simulink library "F3M_aqueousLib"  (R2023b)
settings: Solver=VariableStepAuto  StartTime=0.0  StopTime=10.0  RelTol=1e-3
undefined symbols (not defined in the file): entity, F3_getArrayPos, F3_ptableToFlow, F3_ptableToGain, IAT_flowOut, updateInventoryAndEntity
libraries: F3M_commonLib x1
settings Model: Creator=nshoman  LastModifiedBy=nshoman

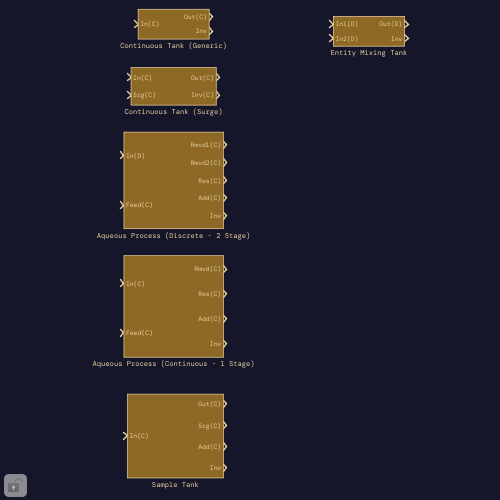
[thumbnail: Simulink's stored preview of the top-level diagram]
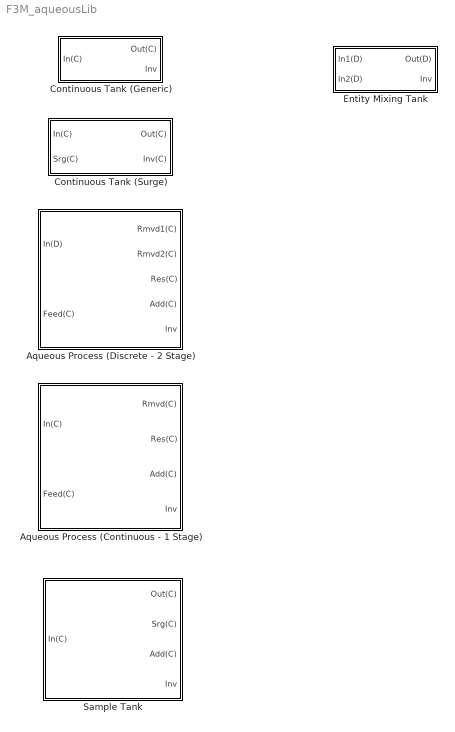
== system F3M_aqueousLib ==
  Aqueous Process (Continuous - 1 Stage) : Subsystem  mask(Aqueous Process (Continuous - 1 Stage)){flowSpecies=at1, flowOut=0, ssOutCB=off, processMn=0, processMx=0, ptable={}, ptable2={}}
      mask prompts: flowSpecies "Process basis"; flowOut "Flow out (/hr)"; ssOutCB "Match inflow"; processMn "Process off point"; processMx "Process on point"; ptable "Additions"; ptable2 "Removals"
      mask help: This block belongs to the larger group of aqueous process blocks. Specifically, this continuous - 1 stage block accepts an input signal that is passed through a process stage, and outputs a continuous signal. The user can also specify additional materials to add to the process, either using the Feed(C) inport or by specifying species in the additions dialog table. If the dialog table is used, material is only added when entities arrive. The Add(C) output provides a signal that describes material that is added by the dialog table, if used.
      mask TypeOptions flowSpecies: at1
      mask Callback ssOutCB:
      | maskStr = get_param(gcb,'ssOutCB');
      | 
      |     if strcmp(maskStr,'on')
      |         set_param(gcb,'MaskEnables',{'on';'off';'on';'on';'on';'on';'on'})
      |     else
      |        set_param(gcb,'MaskEnables',{'on';'on';'on';'on';'on';'on';'on'})
      |     end
      mask DialogControl addCC Prompt: Add species
      mask DialogControl addCC Callback:
      | maskObj = Simulink.Mask.get(gcb);
      |     tableControl = maskObj.getDialogControl('ptable');
      |     tableControl.addRow('a','b')
      mask DialogControl removeCC Prompt: Remove species
      mask DialogControl removeCC Callback:
      | maskObj = Simulink.Mask.get(gcb);
      |     tableControl = maskObj.getDialogControl('ptable');
      |     nrow = tableControl.getNumberOfRows();
      |     if nrow>0
      |         tableControl.removeRow(nrow);
      |     end
      mask DialogControl addOG Prompt: Add species
      mask DialogControl addOG Callback:
      | maskObj = Simulink.Mask.get(gcb);
      |     tableControl = maskObj.getDialogControl('ptable2');
      |     tableControl.addRow('a','b')
      mask DialogControl removeOG Prompt: Remove species
      mask DialogControl removeOG Callback:
      | maskObj = Simulink.Mask.get(gcb);
      |     tableControl = maskObj.getDialogControl('ptable2');
      |     nrow = tableControl.getNumberOfRows();
      |     if nrow>0
      |         tableControl.removeRow(nrow);
      |     end
  Aqueous Process (Discrete - 2 Stage) : Subsystem  mask(Aqueous Process (Discrete - 2 Stage)){flowSpecies=at1, flowOut=5, ssOutCB=off, processMn=0, processMx=0, ptable3={}, ptable={}, ptable2={}}
      mask prompts: flowSpecies "Process basis"; flowOut "Flow out (/hr)"; ssOutCB "Match inflow"; processMn "Process off point"; processMx "Process on point"; ptable3 "Additions"; ptable "Stage 1"; ptable2 "Stage 2"
      mask help: This block belongs to the larger group of aqueous process blocks. Specifically, this discrete - 2 stage blocks accepts an input entity, converts it to a signal, passes the signal through a maximum of two sequential stages, and outputs a continuous signal. The user can also specify additional materials to add to the process, either using the Feed(C) inport or by specifying species in the additions dialog table. If the dialog table is used, material is only added when entities arrive. The Add(C) output provides a signal that describes material that is added by the dialog table, if used.
      mask TypeOptions flowSpecies: at1
      mask Callback ssOutCB:
      | maskStr = get_param(gcb,'ssOutCB');
      | 
      |     if strcmp(maskStr,'on')
      |         set_param(gcb,'MaskEnables',{'on';'off';'on';'on';'on';'on';'on';'on'})
      |     else
      |        set_param(gcb,'MaskEnables',{'on';'on';'on';'on';'on';'on';'on';'on'})
      |     end
      mask DialogControl addCC Prompt: Add species
      mask DialogControl addCC Callback:
      | maskObj = Simulink.Mask.get(gcb);
      |     tableControl = maskObj.getDialogControl('ptable3');
      |     tableControl.addRow('a','b')
      mask DialogControl removeCC Prompt: Remove species
      mask DialogControl removeCC Callback:
      | maskObj = Simulink.Mask.get(gcb);
      |     tableControl = maskObj.getDialogControl('ptable3');
      |     nrow = tableControl.getNumberOfRows();
      |     if nrow>0
      |         tableControl.removeRow(nrow);
      |     end
      mask DialogControl Container3 Prompt: Efficiencies
      mask DialogControl addOG Prompt: Add species
      mask DialogControl addOG Callback:
      | maskObj = Simulink.Mask.get(gcb);
      |     tableControl = maskObj.getDialogControl('ptable');
      |     tableControl.addRow('a','b')
      mask DialogControl removeOG Prompt: Remove species
      mask DialogControl removeOG Callback:
      | maskObj = Simulink.Mask.get(gcb);
      |     tableControl = maskObj.getDialogControl('ptable');
      |     nrow = tableControl.getNumberOfRows();
      |     if nrow>0
      |         tableControl.removeRow(nrow);
      |     end
      mask DialogControl addH Prompt: Add species
      mask DialogControl addH Callback:
      | maskObj = Simulink.Mask.get(gcb);
      |     tableControl = maskObj.getDialogControl('ptable2');
      |     tableControl.addRow('a','b')
      mask DialogControl removeH Prompt: Remove species
      mask DialogControl removeH Callback:
      | maskObj = Simulink.Mask.get(gcb);
      |     tableControl = maskObj.getDialogControl('ptable2');
      |     nrow = tableControl.getNumberOfRows();
      |     if nrow>0
      |         tableControl.removeRow(nrow);
      |     end
  Continuous Tank (Generic) : Subsystem  mask(Continuous Tank (Generic)){isoelelevel=at1, tmin=0, tmax=0, sflowrate=off, flow=0}
      mask prompts: isoelelevel "Tank level basis"; tmin "Tank off point (kg)"; tmax "Tank on point (kg)"; sflowrate "Match inflow"; flow "Flowrate (kg/hr)"
      mask help: The generic continuous tank models a tank that fills and empties based on user specified criteria.
      mask TypeOptions isoelelevel: at1
      mask Callback sflowrate:
      | maskStr = get_param(gcb,'sflowrate');
      | 
      |     if strcmp(maskStr,'on')
      |         set_param(gcb,'MaskEnables',{'on';'on';'on';'on';'off'})
      |     else
      |        set_param(gcb,'MaskEnables',{'on';'on';'on';'on';'on'})
      |     end
  Continuous Tank (Surge) : Subsystem  mask(The generic continuous tank models a tank that fills and empties based on user specified criteria.){isoelelevel=h, tmin=0, tmax=0, sflowrate=off, flow=0}
      mask prompts: isoelelevel "Tank level basis"; tmin "Tank min level (kg)"; tmax "Tank max level (kg)"; sflowrate "Specific flow rate out?"; flow "Flowrate (kg/hr)"
      mask help: This surge continuous models a tank that fills and empties based on user specified criteria and an external surge signal. For this tank to output, both the tank setpoints (i.e., tank on and off points) must be met and the surge signal must be on.
      mask TypeOptions isoelelevel: h
      mask Callback sflowrate:
      | maskStr = get_param(gcb,'sflowrate');
      | 
      |     if strcmp(maskStr,'on')
      |         set_param(gcb,'MaskEnables',{'on';'on';'on';'on';'on'})
      |     else
      |        set_param(gcb,'MaskEnables',{'on';'on';'on';'on';'off'})
      |     end
  Entity Mixing Tank : Subsystem  mask(Entity Mixing Tank){tprocess=0}
      mask prompts: tprocess "Processing time (hr)"
      mask help: This block simulates the mixing of two entities into one. A hold time can be specified to simulate processing time.
  Sample Tank : Subsystem  mask(Sample Tank){species=at1, tMin=0, tMax=0, flowOut=0, delayT=0, ptable={}}
      mask prompts: species "Tank level basis"; tMin "Tank off point"; tMax "Tank on point"; flowOut "Flowrate (kg/hr)"; delayT "Sample time (hr)"; ptable "Material additions"
      mask help: The sample tank simulates the sampling of a material flow. Specifically, this block fills, holds material for a specified amount of time, then empties. The user can optionally specify additional material that should be added when the inflow is non-zero (i.e., material is arriving at this block).
      mask TypeOptions species: at1
      mask DialogControl addS Prompt: Add species
      mask DialogControl addS Callback:
      | maskObj = Simulink.Mask.get(gcb);
      |     tableControl = maskObj.getDialogControl('ptable');
      |     tableControl.addRow('a','b')
      mask DialogControl removeS Prompt: Remove species
      mask DialogControl removeS Callback:
      | maskObj = Simulink.Mask.get(gcb);
      |     tableControl = maskObj.getDialogControl('ptable');
      |     nrow = tableControl.getNumberOfRows();
      |     if nrow>0
      |         tableControl.removeRow(nrow);
      |     end

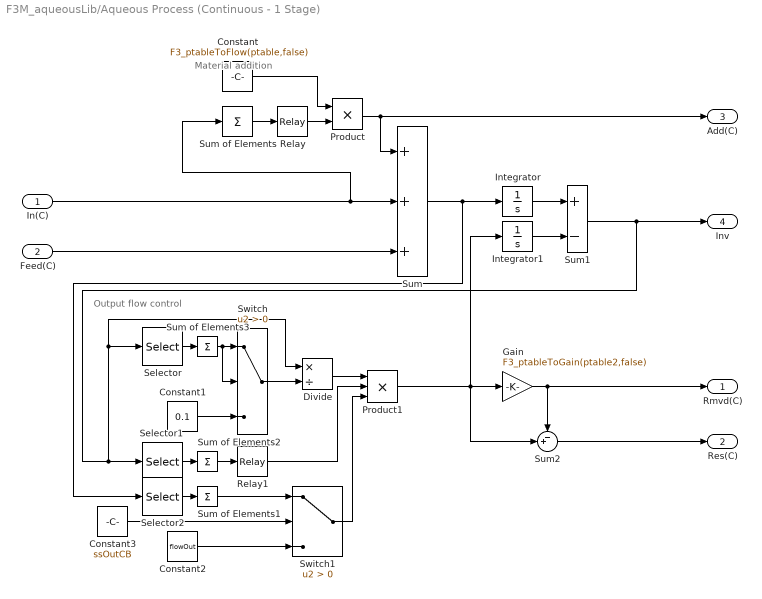
== system F3M_aqueousLib/Aqueous Process (Continuous - 1 Stage) ==
  note: Output flow control
  note: Material addition
  In(C) : Inport
  Feed(C) : Inport  Port=2
  Constant : Constant  Value=F3_ptableToFlow(ptable,false)
  Constant1 : Constant  Value=0.1
  Constant2 : Constant  Value=flowOut
  Constant3 : Constant  Value=ssOutCB
  Divide : Product  Inputs=*/
  Gain : Gain  Gain=F3_ptableToGain(ptable2,false)
  Integrator : Integrator
  Integrator1 : Integrator
  Product : Product
  Product1 : Product  Inputs=3
  Relay : Relay
  Relay1 : Relay  OnSwitchValue=processMx  OffSwitchValue=processMn
  Selector : Selector  InputPortWidth=1677  IndexOptions=Index vector (dialog)  Indices=F3_getArrayPos(flowSpecies)  OutputSizes=1
  Selector1 : Selector  InputPortWidth=1677  IndexOptions=Index vector (dialog)  Indices=F3_getArrayPos(flowSpecies)  OutputSizes=1
  Selector2 : Selector  InputPortWidth=1677  IndexOptions=Index vector (dialog)  Indices=F3_getArrayPos(flowSpecies)  OutputSizes=1
  Sum : Sum  Inputs=+++
  Sum of Elements{,1..3} (4 alike) : Sum  Inputs=+
  Sum1 : Sum  Inputs=+-
  Sum2 : Sum  Inputs=-+|
  Switch : Switch  Criteria=u2 > Threshold  SaturateOnIntegerOverflow=off  InputSameDT=off
  Switch1 : Switch  Criteria=u2 > Threshold  SaturateOnIntegerOverflow=off  InputSameDT=off
  Rmvd(C) : Outport
  Res(C) : Outport  Port=2
  Add(C) : Outport  Port=3
  Inv : Outport  Port=4
  wires:
  Integrator/1 -> Sum1/1
  Product/1 -> Sum/1, Add(C)/1
  Constant/1 -> Product/1
  Sum of Elements/1 -> Relay/1
  Product1/1 -> Sum2/2, Gain/1, Integrator1/1
  Relay/1 -> Product/2
  In(C)/1 -> Sum of Elements/1, Sum/2
  Gain/1 -> Rmvd(C)/1, Sum2/1
  Sum1/1 -> Inv/1, Divide/1, Selector/1, Selector1/1
  Switch/1 -> Divide/2
  Integrator1/1 -> Sum1/2
  Divide/1 -> Product1/1
  Sum/1 -> Selector2/1, Integrator/1
  Constant1/1 -> Switch/3
  Feed(C)/1 -> Sum/3
  Sum2/1 -> Res(C)/1
  Relay1/1 -> Product1/2
  Constant2/1 -> Switch1/3
  Switch1/1 -> Product1/3
  Constant3/1 -> Switch1/2
  Selector2/1 -> Sum of Elements1/1
  Sum of Elements1/1 -> Switch1/1
  Selector1/1 -> Sum of Elements2/1
  Sum of Elements2/1 -> Relay1/1
  Selector/1 -> Sum of Elements3/1
  Sum of Elements3/1 -> Switch/2, Switch/1

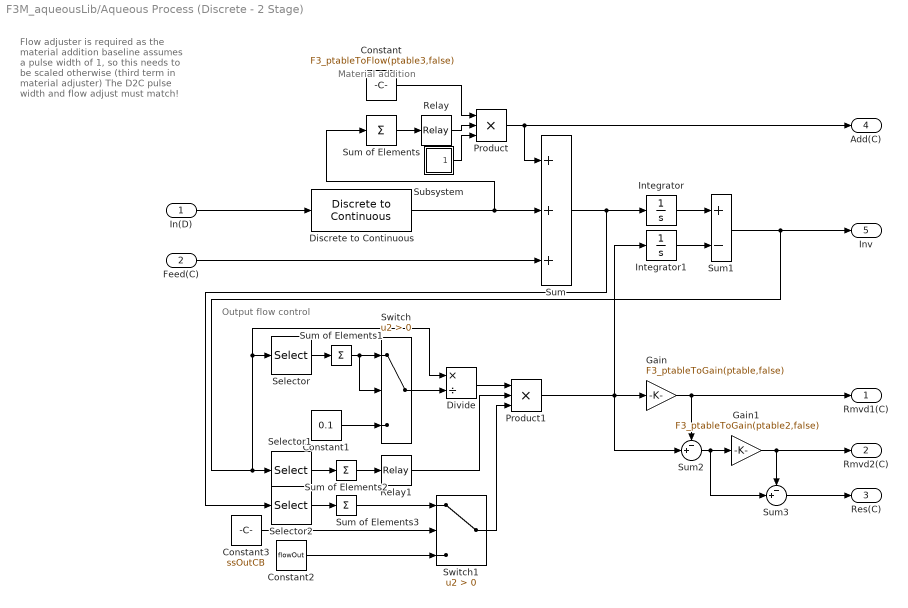
== system F3M_aqueousLib/Aqueous Process (Discrete - 2 Stage) ==
  note: Flow adjuster is
      | required as the material
      | addition baseline assumes
      | a pulse width of 1, so
      | this needs to be scaled
      | otherwise (third term in
      | material adjuster)
      |
      | The D2C pulse width and
      | flow adjust must match!
  note: Material addition
  note: Output flow control
  In(D) : Inport
  Feed(C) : Inport  Port=2
  Constant : Constant  Value=F3_ptableToFlow(ptable3,false)
  Constant1 : Constant  Value=0.1
  Constant2 : Constant  Value=flowOut
  Constant3 : Constant  Value=ssOutCB
  Discrete to Continuous : F3M_commonLib/Discrete to Continuous  width=eps
      settings: SourceProductName=Fissile Facility Flow Modeler
  Divide : Product  Inputs=*/
  Gain : Gain  Gain=F3_ptableToGain(ptable,false)
  Gain1 : Gain  Gain=F3_ptableToGain(ptable2,false)
  Integrator : Integrator
  Integrator1 : Integrator
  Product : Product  Inputs=3
  Product1 : Product  Inputs=3
  Relay : Relay
  Relay1 : Relay  OnSwitchValue=processMx  OffSwitchValue=processMn
  Selector : Selector  InputPortWidth=1677  IndexOptions=Index vector (dialog)  Indices=F3_getArrayPos(flowSpecies)  OutputSizes=1
  Selector1 : Selector  InputPortWidth=1677  IndexOptions=Index vector (dialog)  Indices=F3_getArrayPos(flowSpecies)  OutputSizes=1
  Selector2 : Selector  InputPortWidth=1677  IndexOptions=Index vector (dialog)  Indices=F3_getArrayPos(flowSpecies)  OutputSizes=1
  Subsystem : Subsystem  mask{width=eps}
      mask prompts: width "D2C Pulse Width"
      mask init:
      | mask_parameters = Simulink.Mask.get(gcb);
      | width_value = '';
      | for i = 1:length(mask_parameters.Parameters)
      |     if strcmp(mask_parameters.Parameters(i).Name, 'width')
      |         width_value = mask_parameters.Parameters(i).Value;
      |         break;
      |     end
      | end    
      | if strcmp(width_value, "eps")
      |     %width_internal = str2double(get_param(bdroot(),'MaxStep'));
      |     width_internal = 0.05;
      | else
      |     width_internal = str2double(width_value);
      | end
      mask Callback width:
      | mask_parameters = Simulink.Mask.get(gcb);
      | width_value = '';
      | for i = 1:length(mask_parameters.Parameters)
      |     if strcmp(mask_parameters.Parameters(i).Name, 'width')
      |         width_value = mask_parameters.Parameters(i).Value;
      |         break;
      |     end
      | end
      | if strcmp(width_value, "eps")
      |         %width_internal = str2double(get_param(bdroot(),'MaxStep'));
      |         width_internal = 0.05;
      | else
      |     width_internal = str2double(width_value);
      | end
  Sum : Sum  Inputs=+++
  Sum of Elements{,1..3} (4 alike) : Sum  Inputs=+
  Sum1 : Sum  Inputs=+-
  Sum2 : Sum  Inputs=-+|
  Sum3 : Sum  Inputs=-+|
  Switch : Switch  Criteria=u2 > Threshold  SaturateOnIntegerOverflow=off  InputSameDT=off
  Switch1 : Switch  Criteria=u2 > Threshold  SaturateOnIntegerOverflow=off  InputSameDT=off
  Rmvd1(C) : Outport
  Rmvd2(C) : Outport  Port=2
  Res(C) : Outport  Port=3
  Add(C) : Outport  Port=4
  Inv : Outport  Port=5
  wires:
  In(D)/1 -> Discrete to Continuous/1
  Discrete to Continuous/1 -> Sum of Elements/1, Sum/2
  Feed(C)/1 -> Sum/3
  Sum of Elements/1 -> Relay/1
  Relay/1 -> Product/2
  Product/1 -> Add(C)/1, Sum/1
  Constant/1 -> Product/1
  Sum/1 -> Selector2/1, Integrator/1
  Integrator/1 -> Sum1/1
  Sum1/1 -> Inv/1, Divide/1, Selector/1, Selector1/1
  Selector/1 -> Sum of Elements1/1
  Constant1/1 -> Switch/3
  Switch/1 -> Divide/2
  Divide/1 -> Product1/1
  Selector1/1 -> Sum of Elements2/1
  Product1/1 -> Sum2/2, Gain/1, Integrator1/1
  Gain/1 -> Rmvd1(C)/1, Sum2/1
  Sum2/1 -> Sum3/2, Gain1/1
  Gain1/1 -> Rmvd2(C)/1, Sum3/1
  Integrator1/1 -> Sum1/2
  Sum3/1 -> Res(C)/1
  Relay1/1 -> Product1/2
  Constant2/1 -> Switch1/3
  Switch1/1 -> Product1/3
  Constant3/1 -> Switch1/2
  Sum of Elements2/1 -> Relay1/1
  Sum of Elements1/1 -> Switch/2, Switch/1
  Selector2/1 -> Sum of Elements3/1
  Sum of Elements3/1 -> Switch1/1
  Subsystem/1(Out1) -> Product/3

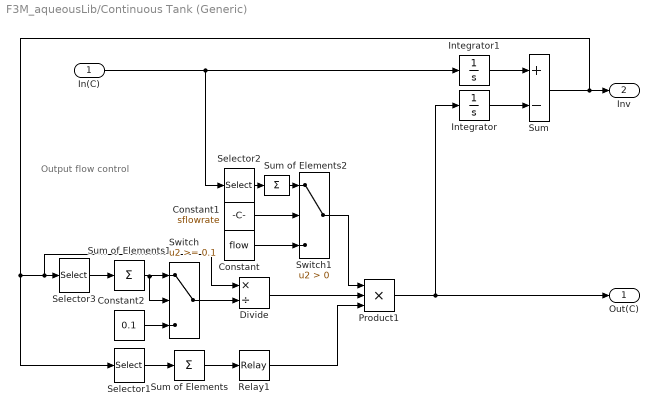
== system F3M_aqueousLib/Continuous Tank (Generic) ==
  note: Output flow control
  In(C) : Inport
  Constant : Constant  Value=flow
  Constant1 : Constant  Value=sflowrate
  Constant2 : Constant  Value=0.1
  Divide : Product  Inputs=*/
  Integrator : Integrator
  Integrator1 : Integrator
  Product1 : Product  Inputs=3
  Relay1 : Relay  OnSwitchValue=tmax  OffSwitchValue=tmin
  Selector1 : Selector  InputPortWidth=1677  IndexOptions=Index vector (dialog)  Indices=F3_getArrayPos(isoelelevel)  OutputSizes=1
  Selector2 : Selector  InputPortWidth=1677  IndexOptions=Index vector (dialog)  Indices=F3_getArrayPos(isoelelevel)  OutputSizes=1
  Selector3 : Selector  InputPortWidth=1677  IndexOptions=Index vector (dialog)  Indices=F3_getArrayPos(isoelelevel)  OutputSizes=1
  Sum : Sum  Inputs=+-
  Sum of Elements : Sum  Inputs=+
  Sum of Elements1 : Sum  Inputs=+
  Sum of Elements2 : Sum  Inputs=+
  Switch : Switch  Threshold=0.1  SaturateOnIntegerOverflow=off  InputSameDT=off
  Switch1 : Switch  Criteria=u2 > Threshold  SaturateOnIntegerOverflow=off  InputSameDT=off
  Out(C) : Outport
  Inv : Outport  Port=2
  wires:
  Constant2/1 -> Switch/3
  Relay1/1 -> Product1/3
  Selector1/1 -> Sum of Elements/1
  Switch/1 -> Divide/2
  Divide/1 -> Product1/2
  Switch1/1 -> Product1/1
  Constant/1 -> Switch1/3
  Constant1/1 -> Switch1/2
  Sum/1 -> Selector1/1, Divide/1, Selector3/1, Inv/1
  Integrator/1 -> Sum/2
  Integrator1/1 -> Sum/1
  In(C)/1 -> Selector2/1, Integrator1/1
  Product1/1 -> Out(C)/1, Integrator/1
  Sum of Elements/1 -> Relay1/1
  Selector3/1 -> Sum of Elements1/1
  Sum of Elements1/1 -> Switch/1, Switch/2
  Selector2/1 -> Sum of Elements2/1
  Sum of Elements2/1 -> Switch1/1

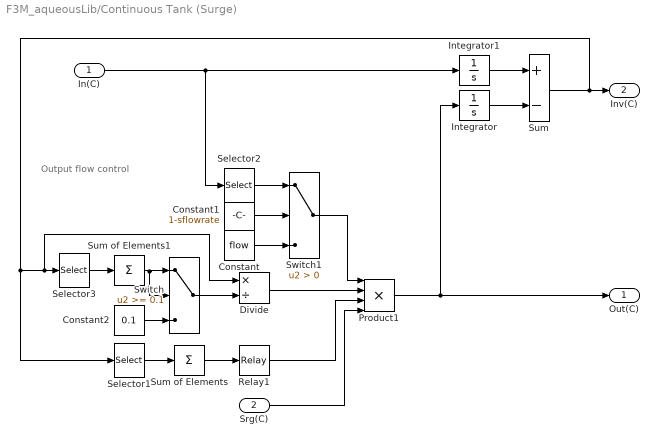
== system F3M_aqueousLib/Continuous Tank (Surge) ==
  note: Output flow control
  In(C) : Inport
  Srg(C) : Inport  Port=2
  Constant : Constant  Value=flow
  Constant1 : Constant  Value=1-sflowrate
  Constant2 : Constant  Value=0.1
  Divide : Product  Inputs=*/
  Integrator : Integrator
  Integrator1 : Integrator
  Product1 : Product  Inputs=4
  Relay1 : Relay  OnSwitchValue=tmax  OffSwitchValue=tmin
  Selector1 : Selector  InputPortWidth=1677  IndexOptions=Index vector (dialog)  Indices=F3_getArrayPos(isoelelevel)  OutputSizes=1
  Selector2 : Selector  InputPortWidth=1677  IndexOptions=Index vector (dialog)  Indices=F3_getArrayPos(isoelelevel)  OutputSizes=1
  Selector3 : Selector  InputPortWidth=1677  IndexOptions=Index vector (dialog)  Indices=F3_getArrayPos(isoelelevel)  OutputSizes=1
  Sum : Sum  Inputs=+-
  Sum of Elements : Sum  Inputs=+
  Sum of Elements1 : Sum  Inputs=+
  Switch : Switch  Threshold=0.1  SaturateOnIntegerOverflow=off  InputSameDT=off
  Switch1 : Switch  Criteria=u2 > Threshold  SaturateOnIntegerOverflow=off  InputSameDT=off
  Out(C) : Outport
  Inv(C) : Outport  Port=2
  wires:
  Divide/1 -> Product1/2
  Sum/1 -> Selector1/1, Divide/1, Selector3/1, Inv(C)/1
  Constant2/1 -> Switch/3
  Switch1/1 -> Product1/1
  Constant1/1 -> Switch1/2
  Switch/1 -> Divide/2
  Selector3/1 -> Sum of Elements1/1
  In(C)/1 -> Selector2/1, Integrator1/1
  Selector2/1 -> Switch1/1
  Constant/1 -> Switch1/3
  Selector1/1 -> Sum of Elements/1
  Relay1/1 -> Product1/3
  Sum of Elements/1 -> Relay1/1
  Integrator/1 -> Sum/2
  Sum of Elements1/1 -> Switch/2, Switch/1
  Integrator1/1 -> Sum/1
  Srg(C)/1 -> Product1/4
  Product1/1 -> Out(C)/1, Integrator/1

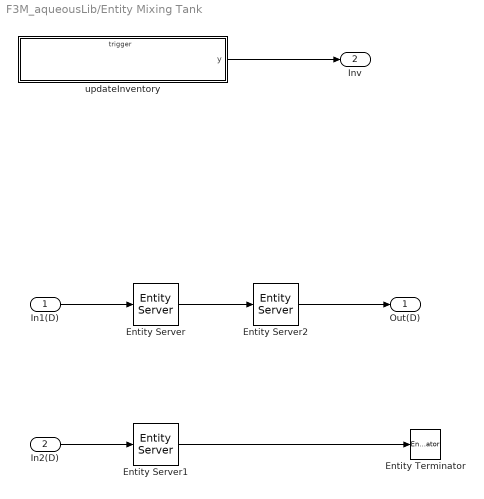
== system F3M_aqueousLib/Entity Mixing Tank ==
  In1(D) : Inport
  In2(D) : Inport  Port=2
  Entity Server : EntityServer  InputPortMessageModes=m  OutputPortMessageModes=m  Capacity=1  ServiceTimeValue=0  EntryAction=entity.isovec = updateInventoryAndEntity(entity.isovec,1);
  Entity Server1 : EntityServer  InputPortMessageModes=m  OutputPortMessageModes=m  Capacity=1  ServiceTimeValue=0  ServiceCompleteAction=updateInventoryAndEntity(entity.isovec,1);
  Entity Server2 : EntityServer  InputPortMessageModes=m  OutputPortMessageModes=m  Capacity=1  ServiceTimeValue=tprocess  ServiceCompleteAction=entity.isovec = updateInventoryAndEntity(entity.isovec,-1);
  Entity Terminator : EntityTerminator  InputPortMessageModes=m
  updateInventory : Subsystem  TreatAsAtomicUnit=on
  Out(D) : Outport
  Inv : Outport  Port=2
  wires:
  In1(D)/1 -> Entity Server/1
  updateInventory/1(y) -> Inv/1
  In2(D)/1 -> Entity Server1/1
  Entity Server1/1 -> Entity Terminator/1
  Entity Server2/1 -> Out(D)/1
  Entity Server/1 -> Entity Server2/1

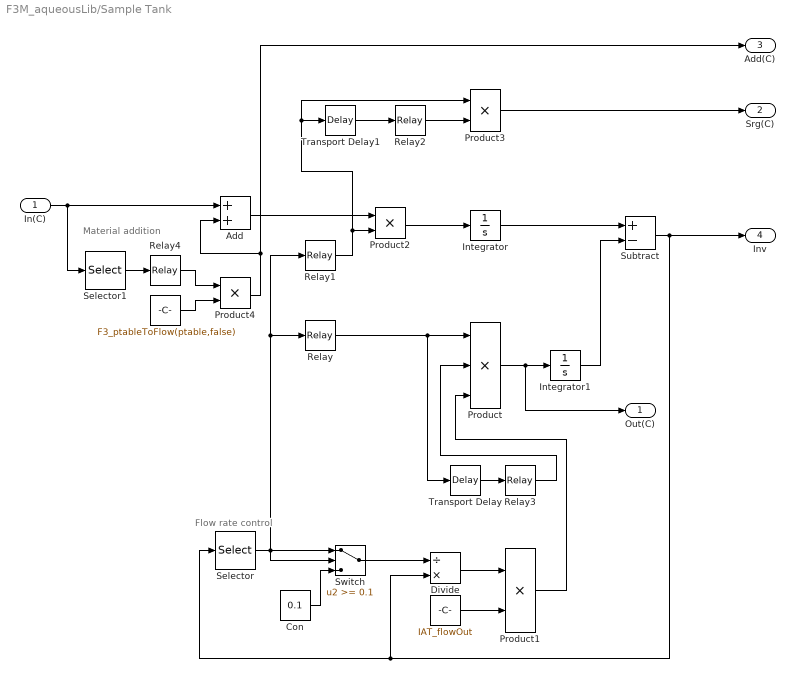
== system F3M_aqueousLib/Sample Tank ==
  note: Material addition
  note: Flow rate control
  In(C) : Inport
  " " : Constant  Value=F3_ptableToFlow(ptable,false)
  "  " : Constant  Value=IAT_flowOut
  Add : Sum
  Con : Constant  Value=0.1
  Divide : Product  Inputs=/*
  Integrator : Integrator
  Integrator1 : Integrator
  Product : Product  Inputs=3  RndMeth=Zero
  Product{1..4} (4 alike) : Product  RndMeth=Zero
  Relay : Relay  OnSwitchValue=tMax  OffSwitchValue=tMin
  Relay1 : Relay  OnSwitchValue=tMax  OffSwitchValue=tMin  OnOutputValue=0  OffOutputValue=1
  Relay2 : Relay  OnSwitchValue=1  OffSwitchValue=0
  Relay3 : Relay  OnSwitchValue=1  OffSwitchValue=0
  Relay4 : Relay  OnSwitchValue=0.01  OffSwitchValue=0
  Selector : Selector  InputPortWidth=1677  IndexOptions=Index vector (dialog)  Indices=[1676]  OutputSizes=1
  Selector1 : Selector  InputPortWidth=1677  IndexOptions=Index vector (dialog)  Indices=[1676]  OutputSizes=1
  Subtract : Sum  Inputs=+-
  Switch : Switch  Threshold=0.1  SaturateOnIntegerOverflow=off  InputSameDT=off
  Transport Delay : TransportDelay  DelayTime=delayT
  Transport Delay1 : TransportDelay  DelayTime=delayT
  Out(C) : Outport  VectorParamsAs1DForOutWhenUnconnected=off
  Srg(C) : Outport  Port=2  VectorParamsAs1DForOutWhenUnconnected=off
  Add(C) : Outport  Port=3  VectorParamsAs1DForOutWhenUnconnected=off
  Inv : Outport  Port=4  VectorParamsAs1DForOutWhenUnconnected=off
  wires:
  Subtract/1 -> Inv/1, Divide/2, Selector/1
  Integrator/1 -> Subtract/1
  Transport Delay/1 -> Relay3/1
  Product2/1 -> Integrator/1
  Product4/1 -> Add(C)/1, Add/2
  Relay/1 -> Transport Delay/1, Product/1
  Relay4/1 -> Product4/1
  Relay1/1 -> Product3/1, Transport Delay1/1, Product2/2
  Product/1 -> Integrator1/1, Out(C)/1
  Selector/1 -> Switch/1, Relay/1, Relay1/1, Switch/2
  "  "/1 -> Product1/2
  " "/1 -> Product4/2
  Add/1 -> Product2/1
  In(C)/1 -> Selector1/1, Add/1
  Selector1/1 -> Relay4/1
  Integrator1/1 -> Subtract/2
  Product3/1 -> Srg(C)/1
  Divide/1 -> Product1/1
  Con/1 -> Switch/3
  Transport Delay1/1 -> Relay2/1
  Product1/1 -> Product/3
  Relay3/1 -> Product/2
  Relay2/1 -> Product3/2
  Switch/1 -> Divide/1

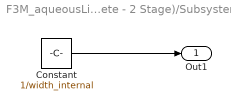
== system F3M_aqueousLib/Aqueous Process (Discrete - 2 Stage)/Subsystem ==
  Constant : Constant  Value=1/width_internal
  Out1 : Outport
  wires:
  Constant/1 -> Out1/1

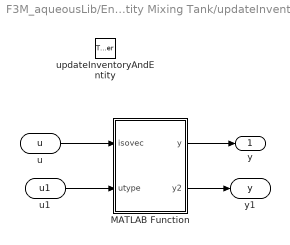
== system F3M_aqueousLib/Entity Mixing Tank/updateInventory ==
  updateInventoryAndEntity : TriggerPort  TriggerType=function-call  IsSimulinkFunction=on  FunctionName=updateInventoryAndEntity  FunctionVisibility=scoped  VariantControl=(inherit)
  MATLAB Function : MATLAB Function  TreatAsAtomicUnit=on
  u : ArgIn  DisableCoverage=on  PortDimensions=1677  ArgumentName=u
  u1 : ArgIn  DisableCoverage=on  Port=2  ArgumentName=u1
  y1 : ArgOut  DisableCoverage=on  PortDimensions=1677  ArgumentName=y
  y : Outport
  wires:
  u/1 -> MATLAB Function/1(isovec)
  u1/1 -> MATLAB Function/2(utype)
  MATLAB Function/1(y) -> y/1
  MATLAB Function/2(y2) -> y1/1

== matlab function F3M_aqueousLib/Entity Mixing Tank/updateInventory/MATLAB Function ==
  data: isovec input; y output; utype input; y2 output
function [y,y2]= fcn(isovec, utype)

persistent inventory


if isempty(inventory)
    inventory = isovec;
else
    if utype == 1 
        inventory = inventory+isovec;
    else 
        isovec = inventory;
        inventory = inventory-isovec;
    end
end




y = inventory;
y2 = isovec;
